simulink model "p_11"  (R2018b)
settings: Solver=VariableStepAuto  StartTime=0.0  StopTime=50  MaxStep=0.01  RelTol=1e-3
settings Model: Creator=kekos  LastModifiedBy=kekos

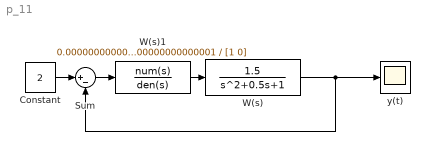
== system p_11 ==
  Constant : Constant  Value=2
  Sum : Sum  Inputs=|+-
  W(s) : TransferFcn  Numerator=[1.5]  Denominator=[1 0.5 1]
  W(s)1 : TransferFcn  Numerator=0.000000000000000000000000001  Denominator=[1 0]
  y(t) : Scope
  wires:
  W(s)1/1 -> W(s)/1
  Sum/1 -> W(s)1/1
  W(s)/1 -> y(t)/1, Sum/2
  Constant/1 -> Sum/1
